simulink model "linearizzazione_feedback"  (R2022b)
settings: Solver=VariableStepAuto  StartTime=0.0  StopTime=30  FixedStep=0.01  RelTol=1e-3
settings Model: Creator=alexi  LastModifiedBy=alexi

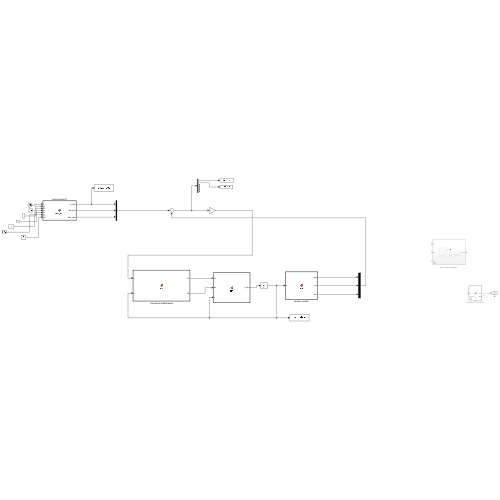
[thumbnail: Simulink's stored preview of the top-level diagram]
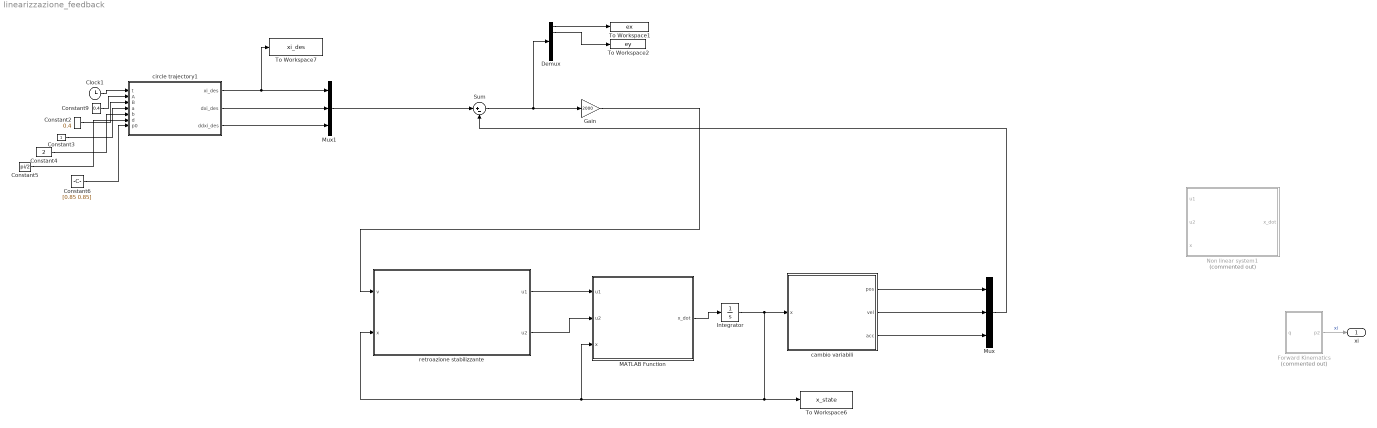
== system linearizzazione_feedback ==
  Clock1 : Clock
  Constant2 : Constant  Value=0.4
  Constant3 : Constant
  Constant4 : Constant  Value=2
  Constant5 : Constant  Value=pi/2
  Constant6 : Constant  Value=[0.85 0.85]
  Constant9 : Constant  Value=0.4
  Demux : Demux  Outputs=6
  Forward Kinematics : MATLAB Function  Commented=on  TreatAsAtomicUnit=on
  Gain : Gain  Gain=2000
  Integrator : Integrator  InitialCondition=[0.25 0.25 0 0 0.25 0.25]'
  MATLAB Function : MATLAB Function  TreatAsAtomicUnit=on
  Mux : Mux  Inputs=3
  Mux1 : Mux  Inputs=3
  Non linear system1 : Subsystem  Commented=on
  Sum : Sum  Inputs=|+-
  To Workspace1 : ToWorkspace  VariableName=ex  SaveFormat=Timeseries  SampleTime=-1
  To Workspace2 : ToWorkspace  VariableName=ey  SaveFormat=Timeseries  SampleTime=-1
  To Workspace6 : ToWorkspace  VariableName=x_state  SaveFormat=Timeseries  SampleTime=-1
  To Workspace7 : ToWorkspace  VariableName=xi_des  SaveFormat=Timeseries  SampleTime=-1
  cambio variabili : MATLAB Function  TreatAsAtomicUnit=on
  circle trajectory1 : MATLAB Function  TreatAsAtomicUnit=on
  retroazione stabilizzante : MATLAB Function  TreatAsAtomicUnit=on
  xi : Outport
  wires:
  Forward Kinematics/1(p2) -> xi/1  "xi"
  Constant4/1 -> circle trajectory1/5(b)
  Constant5/1 -> circle trajectory1/6(d)
  Constant2/1 -> circle trajectory1/3(B)
  Clock1/1 -> circle trajectory1/1(t)
  Constant6/1 -> circle trajectory1/7(p0)
  Constant3/1 -> circle trajectory1/4(a)
  Constant9/1 -> circle trajectory1/2(A)
  Integrator/1 -> MATLAB Function/3(x), retroazione stabilizzante/2(x), To Workspace6/1, cambio variabili/1(x)
  retroazione stabilizzante/1(u1) -> MATLAB Function/1(u1)
  retroazione stabilizzante/2(u2) -> MATLAB Function/2(u2)
  MATLAB Function/1(x_dot) -> Integrator/1
  cambio variabili/1(pos) -> Mux/1
  cambio variabili/2(vel) -> Mux/2
  cambio variabili/3(acc) -> Mux/3
  circle trajectory1/1(xi_des) -> To Workspace7/1, Mux1/1
  circle trajectory1/2(dxi_des) -> Mux1/2
  circle trajectory1/3(ddxi_des) -> Mux1/3
  Mux1/1 -> Sum/1
  Mux/1 -> Sum/2
  Sum/1 -> Demux/1, Gain/1
  Gain/1 -> retroazione stabilizzante/1(v)
  Demux/1 -> To Workspace1/1
  Demux/2 -> To Workspace2/1

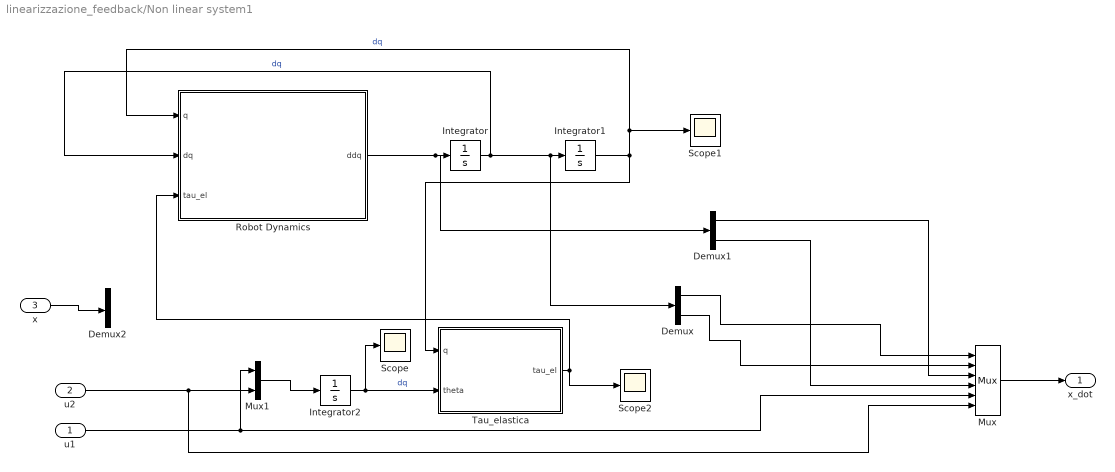
== system linearizzazione_feedback/Non linear system1 ==
  u1 : Inport
  u2 : Inport  Port=2
  x : Inport  Port=3
  Demux : Demux  Outputs=2
  Demux1 : Demux  Outputs=2
  Demux2 : Demux  Outputs=6
  Integrator : Integrator  InitialCondition=[0.25,0.25]'
  Integrator1 : Integrator  InitialCondition=[0.25,0.25]'
  Integrator2 : Integrator  InitialCondition=[0.25 0.25]'
  Mux : Mux  Inputs=6
  Mux1 : Mux  Inputs=2
  Robot Dynamics : MATLAB Function  TreatAsAtomicUnit=on
  Scope : Scope
  Scope1 : Scope
  Scope2 : Scope
  Tau_elastica : Subsystem
  x_dot : Outport
  wires:
  Integrator1/1 -> Tau_elastica/1(q), Scope1/1, Robot Dynamics/1(q)  "dq"
  Integrator/1 -> Robot Dynamics/2(dq), Demux/1, Integrator1/1  "dq"
  Tau_elastica/1(tau_el) -> Scope2/1, Robot Dynamics/3(tau_el)
  Robot Dynamics/1(ddq) -> Demux1/1, Integrator/1
  Demux/1 -> Mux/1
  Demux/2 -> Mux/2
  Demux1/1 -> Mux/3
  Demux1/2 -> Mux/4
  Integrator2/1 -> Scope/1, Tau_elastica/2(theta)  "dq"
  Mux/1 -> x_dot/1
  u1/1 -> Mux1/1, Mux/5
  u2/1 -> Mux1/2, Mux/6
  Mux1/1 -> Integrator2/1
  x/1 -> Demux2/1

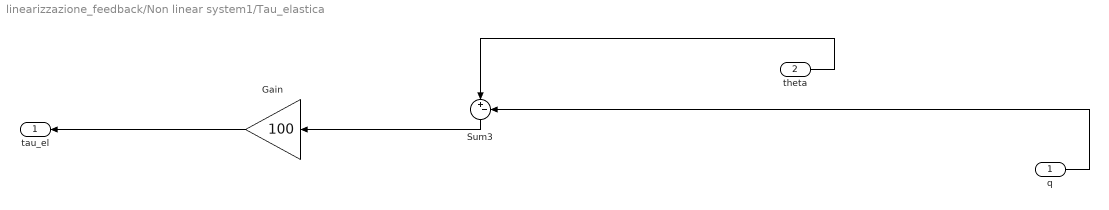
== system linearizzazione_feedback/Non linear system1/Tau_elastica ==
  q : Inport
  theta : Inport  Port=2
  Gain : Gain  Gain=100
  Sum3 : Sum  Inputs=|+-
  tau_el : Outport
  wires:
  Sum3/1 -> Gain/1
  q/1 -> Sum3/2
  Gain/1 -> tau_el/1
  theta/1 -> Sum3/1

== matlab function linearizzazione_feedback/cambio variabili ==
  data: x input; pos output; vel output; acc output
function [pos,vel,acc]= fcn(x)
a1 = 1;
a2 = 1;
k = 10;

q1 = x(1);
q2 = x(2);
dq1 = x(3);
dq2 = x(4);
theta1 = x(5);
theta2 = x(6);

q = [q1;q2];
dq = [dq1;dq2];
theta = [theta1;theta2];
B = RR_mass_matrix(q);
C = RR_coriolis_matrix(q,dq);
G = RR_gravity_vector(q);

% inversa_b = inv(B);
% B11G1 = inversa_b(1,1)*G(1);
% B12G2 = inversa_b(1,2)*G(2);
% B21G1 = inversa_b(2,1)*G(1);
% B22G2 = inversa_b(2,2)*G(2);
% 
% B11C11 = inversa_b(1,1)*C(1,1);
% B12C21 = inversa_b(1,2)*C(2,1);
% B11C12 = inversa_b(1,1)*C(1,2);
% B12C22 = inversa_b(1,2)*C(2,2);
%  
% B21C11 = inversa_b(2,1)*C(1,1);
% B22C21 = inversa_b(2,2)*C(2,1);
% B21C12 = inversa_b(2,1)*C(1,2);
% B22C22 = inversa_b(2,2)*C(2,2);
% 
% b1_1 = inversa_b(1,1);
% b1_2 = inversa_b(1,2);
% b2_1 = inversa_b(2,1);
% b2_2 = inversa_b(2,2);
% 
% c1_1 = C(1,1);
% c1_2 = C(1,2);
% c2_1 = C(2,1);
% c2_2 = C(2,2);
% 
% g1 = G(1);
% g2 = G(2);



% MG1 = MG(1);
% MG2 = MG(2);
% MC = inv(B)*C;
% MC1 = MC(1,1)+MC(1,2);
% MC2 = MC(2,1)+MC(2,2);
% inv = inv(B);
% B1 = inv(1,1) + inv(1,2);
% B2 = inv(2,1) + inv

z1 = a1*cos(q1)+a2*cos(q1+q2); %posizione in x
z2 = -sin(q1)*dq1 - sin(q1+q2)*(dq1+dq2); %derivata prima
%z3 = sin(q1 + q2)*(b1_1*g1 + b1_2*g2 + b2_1*g1 + b2_2*g2 + dq1*(b1_1*c1_1 + b1_2*c2_1) + dq2*(b1_1*c1_2 + b1_2*c2_2) + dq1*(b2_1*c1_1 + b2_2*c2_1) + dq2*(b2_1*c1_2 + b2_2*c2_2) + b1_1*k*(q1 - theta1) + b1_2*k*(q2 - theta2) + b2_1*k*(q1 - theta1) + b2_2*k*(q2 - theta2)) - cos(q1 + q2)*(dq1 + dq2)^2 + sin(q1)*(b1_1*g1 + b1_2*g2 + dq1*(b1_1*c1_1 + b1_2*c2_1) + dq2*(b1_1*c1_2 + b1_2*c2_2) + b1_1*k*(q1 - theta1) + b1_2*k*(q2 - theta2)) - cos(q1)*dq1^2;
z3 = sin(q1)*(dq1*((6*sin(q2)*dq2)/(9*cos(q2)^2 - 16) + (3*sin(q2)*dq1*(3*cos(q2) + 2))/(9*cos(q2)^2 - 16)) - (12*((2943*cos(q1))/200 + (981*cos(q1 + q2))/200))/(9*cos(q2)^2 - 16) - (12*k*(q1 - theta1))/(9*cos(q2)^2 - 16) + (2943*cos(q1 + q2)*(3*cos(q2) + 2))/(100*(9*cos(q2)^2 - 16)) + (6*k*(3*cos(q2) + 2)*(q2 - theta2))/(9*cos(q2)^2 - 16) + (6*sin(q2)*dq2*(dq1 + dq2))/(9*cos(q2)^2 - 16)) - cos(q1 + q2)*(dq1 + dq2)^2 - sin(q1 + q2)*((12*((2943*cos(q1))/200 + (981*cos(q1 + q2))/200))/(9*cos(q2)^2 - 16) - dq1*((6*sin(q2)*dq2)/(9*cos(q2)^2 - 16) + (3*sin(q2)*dq1*(3*cos(q2) + 2))/(9*cos(q2)^2 - 16)) + dq1*((3*sin(q2)*dq2*(3*cos(q2) + 2))/(9*cos(q2)^2 - 16) + (6*sin(q2)*dq1*(3*cos(q2) + 5))/(9*cos(q2)^2 - 16)) + (12*k*(q1 - theta1))/(9*cos(q2)^2 - 16) - (6*(3*cos(q2) + 2)*((2943*cos(q1))/200 + (981*cos(q1 + q2))/200))/(9*cos(q2)^2 - 16) - (2943*cos(q1 + q2)*(3*cos(q2) + 2))/(100*(9*cos(q2)^2 - 16)) + (2943*cos(q1 + q2)*(3*cos(q2) + 5))/(50*(9*cos(q2)^2 - 16)) - (6*k*(3*cos(q2) + 2)*(q1 - theta1))/(9*cos(q2)^2 - 16) - (6*k*(3*cos(q2) + 2)*(q2 - theta2))/(9*cos(q2)^2 - 16) + (12*k*(3*cos(q2) + 5)*(q2 - theta2))/(9*cos(q2)^2 - 16) - (6*sin(q2)*dq2*(dq1 + dq2))/(9*cos(q2)^2 - 16) + (3*sin(q2)*dq2*(3*cos(q2) + 2)*(dq1 + dq2))/(9*cos(q2)^2 - 16)) - cos(q1)*dq1^2;

z4 =  a1*sin(q1)+a2*sin(q1+q2); %posizione in y
z5 = cos(q1)*dq1 + cos(q1+q2)*(dq1+dq2);
%z6 = - cos(q1 + q2)*(b1_1*g1 + b1_2*g2 + b2_1*g1 + b2_2*g2 + dq1*(b1_1*c1_1 + b1_2*c2_1) + dq2*(b1_1*c1_2 + b1_2*c2_2) + dq1*(b2_1*c1_1 + b2_2*c2_1) + dq2*(b2_1*c1_2 + b2_2*c2_2) + b1_1*k*(q1 - theta1) + b1_2*k*(q2 - theta2) + b2_1*k*(q1 - theta1) + b2_2*k*(q2 - theta2)) - sin(q1 + q2)*(dq1 + dq2)^2 - cos(q1)*(b1_1*g1 + b1_2*g2 + dq1*(b1_1*c1_1 + b1_2*c2_1) + dq2*(b1_1*c1_2 + b1_2*c2_2) + b1_1*k*(q1 - theta1) + b1_2*k*(q2 - theta2)) - sin(q1)*dq1^2;
z6 = cos(q1 + q2)*((12*((2943*cos(q1))/200 + (981*cos(q1 + q2))/200))/(9*cos(q2)^2 - 16) - dq1*((6*sin(q2)*dq2)/(9*cos(q2)^2 - 16) + (3*sin(q2)*dq1*(3*cos(q2) + 2))/(9*cos(q2)^2 - 16)) + dq1*((3*sin(q2)*dq2*(3*cos(q2) + 2))/(9*cos(q2)^2 - 16) + (6*sin(q2)*dq1*(3*cos(q2) + 5))/(9*cos(q2)^2 - 16)) + (12*k*(q1 - theta1))/(9*cos(q2)^2 - 16) - (6*(3*cos(q2) + 2)*((2943*cos(q1))/200 + (981*cos(q1 + q2))/200))/(9*cos(q2)^2 - 16) - (2943*cos(q1 + q2)*(3*cos(q2) + 2))/(100*(9*cos(q2)^2 - 16)) + (2943*cos(q1 + q2)*(3*cos(q2) + 5))/(50*(9*cos(q2)^2 - 16)) - (6*k*(3*cos(q2) + 2)*(q1 - theta1))/(9*cos(q2)^2 - 16) - (6*k*(3*cos(q2) + 2)*(q2 - theta2))/(9*cos(q2)^2 - 16) + (12*k*(3*cos(q2) + 5)*(q2 - theta2))/(9*cos(q2)^2 - 16) - (6*sin(q2)*dq2*(dq1 + dq2))/(9*cos(q2)^2 - 16) + (3*sin(q2)*dq2*(3*cos(q2) + 2)*(dq1 + dq2))/(9*cos(q2)^2 - 16)) - cos(q1)*(dq1*((6*sin(q2)*dq2)/(9*cos(q2)^2 - 16) + (3*sin(q2)*dq1*(3*cos(q2) + 2))/(9*cos(q2)^2 - 16)) - (12*((2943*cos(q1))/200 + (981*cos(q1 + q2))/200))/(9*cos(q2)^2 - 16) - (12*k*(q1 - theta1))/(9*cos(q2)^2 - 16) + (2943*cos(q1 + q2)*(3*cos(q2) + 2))/(100*(9*cos(q2)^2 - 16)) + (6*k*(3*cos(q2) + 2)*(q2 - theta2))/(9*cos(q2)^2 - 16) + (6*sin(q2)*dq2*(dq1 + dq2))/(9*cos(q2)^2 - 16)) - sin(q1)*dq1^2 - sin(q1 + q2)*(dq1 + dq2)^2;
pos = [z1;z4];
vel = [z2;z5];
acc = [z3;z6];

== matlab function linearizzazione_feedback/retroazione stabilizzante ==
  data: v input; u1 output; x input; u2 output
function [u1,u2]= fcn(v,x)
k = 10;
q1 = x(1);
q2 = x(2);
dq1 = x(3);
dq2 = x(4);
theta1 = x(5);
theta2 = x(6);

q = [q1;q2];
dq = [dq1;dq2];
B = RR_mass_matrix(q);
C = RR_coriolis_matrix(q,dq);
G = RR_gravity_vector(q);

inversa_b = inv(B);
B11G1 = inversa_b(1,1)*G(1);
B12G2 = inversa_b(1,2)*G(2);
B21G1 = inversa_b(2,1)*G(1);
B22G2 = inversa_b(2,2)*G(2);

B11C11 = inversa_b(1,1)*C(1,1);
B12C21 = inversa_b(1,2)*C(2,1);
B11C12 = inversa_b(1,1)*C(1,2);
B12C22 = inversa_b(1,2)*C(2,2);
 
B21C11 = inversa_b(2,1)*C(1,1);
B22C21 = inversa_b(2,2)*C(2,1);
B21C12 = inversa_b(2,1)*C(1,2);
B22C22 = inversa_b(2,2)*C(2,2);

b1_1 = inversa_b(1,1);
b1_2 = inversa_b(1,2);
b2_1 = inversa_b(2,1);
b2_2 = inversa_b(2,2);

c1_1 = C(1,1);
c1_2 = C(1,2);
c2_1 = C(2,1);
c2_2 = C(2,2);

g1 = G(1);
g2 = G(2);

% x_dtheta1 = - sin(q1 + q2)*(b1_1*k + b2_1*k) - b1_1*k*sin(q1);
% x_dtheta2 = - sin(q1 + q2)*(b1_2*k + b2_2*k) - b1_2*k*sin(q1);
% y_dtheta1 = cos(q1 + q2)*(b1_1*k + b2_1*k) + b1_1*k*cos(q1);
% y_dtheta2 = cos(q1 + q2)*(b1_2*k + b2_2*k) + b1_2*k*cos(q1);

x_dtheta1 = sin(q1 + q2)*((12*k)/(9*cos(q2)^2 - 16) - (6*k*(3*cos(q2) + 2))/(9*cos(q2)^2 - 16)) + (12*k*sin(q1))/(9*cos(q2)^2 - 16);
x_dtheta2 = - sin(q1 + q2)*((6*k*(3*cos(q2) + 2))/(9*cos(q2)^2 - 16) - (12*k*(3*cos(q2) + 5))/(9*cos(q2)^2 - 16)) - (6*k*sin(q1)*(3*cos(q2) + 2))/(9*cos(q2)^2 - 16);
y_dtheta1 = - cos(q1 + q2)*((12*k)/(9*cos(q2)^2 - 16) - (6*k*(3*cos(q2) + 2))/(9*cos(q2)^2 - 16)) - (12*k*cos(q1))/(9*cos(q2)^2 - 16);
y_dtheta2 = cos(q1 + q2)*((6*k*(3*cos(q2) + 2))/(9*cos(q2)^2 - 16) - (12*k*(3*cos(q2) + 5))/(9*cos(q2)^2 - 16)) + (6*k*cos(q1)*(3*cos(q2) + 2))/(9*cos(q2)^2 - 16);

E = [x_dtheta1 x_dtheta2; y_dtheta1 y_dtheta2];
%f_x = sin(q1 + q2)*(dq1 + dq2)^3 - sin(q1)*((b1_1*c1_1 + b1_2*c2_1)*(b1_1*g1 + b1_2*g2 + dq1*(b1_1*c1_1 + b1_2*c2_1) + dq2*(b1_1*c1_2 + b1_2*c2_2) + b1_1*k*(q1 - theta1) + b1_2*k*(q2 - theta2)) + (b1_1*c1_2 + b1_2*c2_2)*(b2_1*g1 + b2_2*g2 + dq1*(b2_1*c1_1 + b2_2*c2_1) + dq2*(b2_1*c1_2 + b2_2*c2_2) + b2_1*k*(q1 - theta1) + b2_2*k*(q2 - theta2)) - b1_1*k*(dq1) - b1_2*k*(dq2)) - sin(q1 + q2)*((b1_1*c1_1 + b1_2*c2_1)*(b1_1*g1 + b1_2*g2 + dq1*(b1_1*c1_1 + b1_2*c2_1) + dq2*(b1_1*c1_2 + b1_2*c2_2) + b1_1*k*(q1 - theta1) + b1_2*k*(q2 - theta2)) + (b2_1*c1_1 + b2_2*c2_1)*(b1_1*g1 + b1_2*g2 + dq1*(b1_1*c1_1 + b1_2*c2_1) + dq2*(b1_1*c1_2 + b1_2*c2_2) + b1_1*k*(q1 - theta1) + b1_2*k*(q2 - theta2)) + (b1_1*c1_2 + b1_2*c2_2)*(b2_1*g1 + b2_2*g2 + dq1*(b2_1*c1_1 + b2_2*c2_1) + dq2*(b2_1*c1_2 + b2_2*c2_2) + b2_1*k*(q1 - theta1) + b2_2*k*(q2 - theta2)) + (b2_1*c1_2 + b2_2*c2_2)*(b2_1*g1 + b2_2*g2 + dq1*(b2_1*c1_1 + b2_2*c2_1) + dq2*(b2_1*c1_2 + b2_2*c2_2) + b2_1*k*(q1 - theta1) + b2_2*k*(q2 - theta2)) - b1_1*k*(dq1) - b1_2*k*(dq2) - b2_1*k*(dq1) - b2_2*k*(dq2)) + sin(q1)*dq1^3 + 3*cos(q1 + q2)*(dq1 + dq2)*(b1_1*g1 + b1_2*g2 + b2_1*g1 + b2_2*g2 + dq1*(b1_1*c1_1 + b1_2*c2_1) + dq2*(b1_1*c1_2 + b1_2*c2_2) + dq1*(b2_1*c1_1 + b2_2*c2_1) + dq2*(b2_1*c1_2 + b2_2*c2_2) + b1_1*k*(q1 - theta1) + b1_2*k*(q2 - theta2) + b2_1*k*(q1 - theta1) + b2_2*k*(q2 - theta2)) + 3*cos(q1)*dq1*(b1_1*g1 + b1_2*g2 + dq1*(b1_1*c1_1 + b1_2*c2_1) + dq2*(b1_1*c1_2 + b1_2*c2_2) + b1_1*k*(q1 - theta1) + b1_2*k*(q2 - theta2));
%f_y = cos(q1)*((b1_1*c1_1 + b1_2*c2_1)*(b1_1*g1 + b1_2*g2 + dq1*(b1_1*c1_1 + b1_2*c2_1) + dq2*(b1_1*c1_2 + b1_2*c2_2) + b1_1*k*(q1 - theta1) + b1_2*k*(q2 - theta2)) + (b1_1*c1_2 + b1_2*c2_2)*(b2_1*g1 + b2_2*g2 + dq1*(b2_1*c1_1 + b2_2*c2_1) + dq2*(b2_1*c1_2 + b2_2*c2_2) + b2_1*k*(q1 - theta1) + b2_2*k*(q2 - theta2)) - b1_1*k*(dq1) - b1_2*k*(dq2)) - cos(q1 + q2)*(dq1 + dq2)^3 + cos(q1 + q2)*((b1_1*c1_1 + b1_2*c2_1)*(b1_1*g1 + b1_2*g2 + dq1*(b1_1*c1_1 + b1_2*c2_1) + dq2*(b1_1*c1_2 + b1_2*c2_2) + b1_1*k*(q1 - theta1) + b1_2*k*(q2 - theta2)) + (b2_1*c1_1 + b2_2*c2_1)*(b1_1*g1 + b1_2*g2 + dq1*(b1_1*c1_1 + b1_2*c2_1) + dq2*(b1_1*c1_2 + b1_2*c2_2) + b1_1*k*(q1 - theta1) + b1_2*k*(q2 - theta2)) + (b1_1*c1_2 + b1_2*c2_2)*(b2_1*g1 + b2_2*g2 + dq1*(b2_1*c1_1 + b2_2*c2_1) + dq2*(b2_1*c1_2 + b2_2*c2_2) + b2_1*k*(q1 - theta1) + b2_2*k*(q2 - theta2)) + (b2_1*c1_2 + b2_2*c2_2)*(b2_1*g1 + b2_2*g2 + dq1*(b2_1*c1_1 + b2_2*c2_1) + dq2*(b2_1*c1_2 + b2_2*c2_2) + b2_1*k*(q1 - theta1) + b2_2*k*(q2 - theta2)) - b1_1*k*(dq1) - b1_2*k*(dq2) - b2_1*k*(dq1) - b2_2*k*(dq2)) - cos(q1)*dq1^3 + 3*sin(q1 + q2)*(dq1 + dq2)*(b1_1*g1 + b1_2*g2 + b2_1*g1 + b2_2*g2 + dq1*(b1_1*c1_1 + b1_2*c2_1) + dq2*(b1_1*c1_2 + b1_2*c2_2) + dq1*(b2_1*c1_1 + b2_2*c2_1) + dq2*(b2_1*c1_2 + b2_2*c2_2) + b1_1*k*(q1 - theta1) + b1_2*k*(q2 - theta2) + b2_1*k*(q1 - theta1) + b2_2*k*(q2 - theta2)) + 3*sin(q1)*dq1*(b1_1*g1 + b1_2*g2 + dq1*(b1_1*c1_1 + b1_2*c2_1) + dq2*(b1_1*c1_2 + b1_2*c2_2) + b1_1*k*(q1 - theta1) + b1_2*k*(q2 - theta2));
f_x = sin(q1 + q2)*(dq1 + dq2)^3 + sin(q1 + q2)*((12*((981*sin(q1 + q2)*(dq1 + dq2))/200 + (2943*sin(q1)*dq1)/200))/(9*cos(q2)^2 - 16) - ((6*sin(q2)*dq2)/(9*cos(q2)^2 - 16) + (3*sin(q2)*dq1*(3*cos(q2) + 2))/(9*cos(q2)^2 - 16))*(dq1*((6*sin(q2)*dq2)/(9*cos(q2)^2 - 16) + (3*sin(q2)*dq1*(3*cos(q2) + 2))/(9*cos(q2)^2 - 16)) - (12*((2943*cos(q1))/200 + (981*cos(q1 + q2))/200))/(9*cos(q2)^2 - 16) - (12*k*(q1 - theta1))/(9*cos(q2)^2 - 16) + (2943*cos(q1 + q2)*(3*cos(q2) + 2))/(100*(9*cos(q2)^2 - 16)) + (6*k*(3*cos(q2) + 2)*(q2 - theta2))/(9*cos(q2)^2 - 16) + (6*sin(q2)*dq2*(dq1 + dq2))/(9*cos(q2)^2 - 16)) + dq1*((6*cos(q2)*dq2^2)/(9*cos(q2)^2 - 16) + (6*sin(q2)*(dq1*((3*sin(q2)*dq2*(3*cos(q2) + 2))/(9*cos(q2)^2 - 16) + (6*sin(q2)*dq1*(3*cos(q2) + 5))/(9*cos(q2)^2 - 16)) - (6*(3*cos(q2) + 2)*((2943*cos(q1))/200 + (981*cos(q1 + q2))/200))/(9*cos(q2)^2 - 16) + (2943*cos(q1 + q2)*(3*cos(q2) + 5))/(50*(9*cos(q2)^2 - 16)) - (6*k*(3*cos(q2) + 2)*(q1 - theta1))/(9*cos(q2)^2 - 16) + (12*k*(3*cos(q2) + 5)*(q2 - theta2))/(9*cos(q2)^2 - 16) + (3*sin(q2)*dq2*(3*cos(q2) + 2)*(dq1 + dq2))/(9*cos(q2)^2 - 16)))/(9*cos(q2)^2 - 16) + (108*cos(q2)*sin(q2)^2*dq2^2)/(9*cos(q2)^2 - 16)^2 - (9*sin(q2)^2*dq1*dq2)/(9*cos(q2)^2 - 16) - (3*sin(q2)*(3*cos(q2) + 2)*(dq1*((6*sin(q2)*dq2)/(9*cos(q2)^2 - 16) + (3*sin(q2)*dq1*(3*cos(q2) + 2))/(9*cos(q2)^2 - 16)) - (12*((2943*cos(q1))/200 + (981*cos(q1 + q2))/200))/(9*cos(q2)^2 - 16) - (12*k*(q1 - theta1))/(9*cos(q2)^2 - 16) + (2943*cos(q1 + q2)*(3*cos(q2) + 2))/(100*(9*cos(q2)^2 - 16)) + (6*k*(3*cos(q2) + 2)*(q2 - theta2))/(9*cos(q2)^2 - 16) + (6*sin(q2)*dq2*(dq1 + dq2))/(9*cos(q2)^2 - 16)))/(9*cos(q2)^2 - 16) + (3*cos(q2)*dq1*dq2*(3*cos(q2) + 2))/(9*cos(q2)^2 - 16) + (54*cos(q2)*sin(q2)^2*dq1*dq2*(3*cos(q2) + 2))/(9*cos(q2)^2 - 16)^2) + ((3*sin(q2)*dq2*(3*cos(q2) + 2))/(9*cos(q2)^2 - 16) + (6*sin(q2)*dq1*(3*cos(q2) + 5))/(9*cos(q2)^2 - 16))*(dq1*((6*sin(q2)*dq2)/(9*cos(q2)^2 - 16) + (3*sin(q2)*dq1*(3*cos(q2) + 2))/(9*cos(q2)^2 - 16)) - (12*((2943*cos(q1))/200 + (981*cos(q1 + q2))/200))/(9*cos(q2)^2 - 16) - (12*k*(q1 - theta1))/(9*cos(q2)^2 - 16) + (2943*cos(q1 + q2)*(3*cos(q2) + 2))/(100*(9*cos(q2)^2 - 16)) + (6*k*(3*cos(q2) + 2)*(q2 - theta2))/(9*cos(q2)^2 - 16) + (6*sin(q2)*dq2*(dq1 + dq2))/(9*cos(q2)^2 - 16)) - dq1*((3*cos(q2)*dq2^2*(3*cos(q2) + 2))/(9*cos(q2)^2 - 16) - (18*sin(q2)^2*dq1*dq2)/(9*cos(q2)^2 - 16) - (6*sin(q2)*(3*cos(q2) + 5)*(dq1*((6*sin(q2)*dq2)/(9*cos(q2)^2 - 16) + (3*sin(q2)*dq1*(3*cos(q2) + 2))/(9*cos(q2)^2 - 16)) - (12*((2943*cos(q1))/200 + (981*cos(q1 + q2))/200))/(9*cos(q2)^2 - 16) - (12*k*(q1 - theta1))/(9*cos(q2)^2 - 16) + (2943*cos(q1 + q2)*(3*cos(q2) + 2))/(100*(9*cos(q2)^2 - 16)) + (6*k*(3*cos(q2) + 2)*(q2 - theta2))/(9*cos(q2)^2 - 16) + (6*sin(q2)*dq2*(dq1 + dq2))/(9*cos(q2)^2 - 16)))/(9*cos(q2)^2 - 16) - (9*sin(q2)^2*dq2^2)/(9*cos(q2)^2 - 16) + (3*sin(q2)*(3*cos(q2) + 2)*(dq1*((3*sin(q2)*dq2*(3*cos(q2) + 2))/(9*cos(q2)^2 - 16) + (6*sin(q2)*dq1*(3*cos(q2) + 5))/(9*cos(q2)^2 - 16)) - (6*(3*cos(q2) + 2)*((2943*cos(q1))/200 + (981*cos(q1 + q2))/200))/(9*cos(q2)^2 - 16) + (2943*cos(q1 + q2)*(3*cos(q2) + 5))/(50*(9*cos(q2)^2 - 16)) - (6*k*(3*cos(q2) + 2)*(q1 - theta1))/(9*cos(q2)^2 - 16) + (12*k*(3*cos(q2) + 5)*(q2 - theta2))/(9*cos(q2)^2 - 16) + (3*sin(q2)*dq2*(3*cos(q2) + 2)*(dq1 + dq2))/(9*cos(q2)^2 - 16)))/(9*cos(q2)^2 - 16) + (6*cos(q2)*dq1*dq2*(3*cos(q2) + 5))/(9*cos(q2)^2 - 16) + (54*cos(q2)*sin(q2)^2*dq2^2*(3*cos(q2) + 2))/(9*cos(q2)^2 - 16)^2 + (108*cos(q2)*sin(q2)^2*dq1*dq2*(3*cos(q2) + 5))/(9*cos(q2)^2 - 16)^2) - (12*k*(dq1))/(9*cos(q2)^2 - 16) - (6*(3*cos(q2) + 2)*((981*sin(q1 + q2)*(dq1 + dq2))/200 + (2943*sin(q1)*dq1)/200))/(9*cos(q2)^2 - 16) + (6*k*(3*cos(q2) + 2)*(dq1))/(9*cos(q2)^2 - 16) + (6*k*(3*cos(q2) + 2)*(dq2))/(9*cos(q2)^2 - 16) - (12*k*(3*cos(q2) + 5)*(dq2))/(9*cos(q2)^2 - 16) + (9*sin(q2)^2*dq2^2*(dq1 + dq2))/(9*cos(q2)^2 - 16) - (18*sin(q2)*dq2*((2943*cos(q1))/200 + (981*cos(q1 + q2))/200))/(9*cos(q2)^2 - 16) + (6*sin(q2)*dq2*((12*((2943*cos(q1))/200 + (981*cos(q1 + q2))/200))/(9*cos(q2)^2 - 16) - dq1*((6*sin(q2)*dq2)/(9*cos(q2)^2 - 16) + (3*sin(q2)*dq1*(3*cos(q2) + 2))/(9*cos(q2)^2 - 16)) + dq1*((3*sin(q2)*dq2*(3*cos(q2) + 2))/(9*cos(q2)^2 - 16) + (6*sin(q2)*dq1*(3*cos(q2) + 5))/(9*cos(q2)^2 - 16)) + (12*k*(q1 - theta1))/(9*cos(q2)^2 - 16) - (6*(3*cos(q2) + 2)*((2943*cos(q1))/200 + (981*cos(q1 + q2))/200))/(9*cos(q2)^2 - 16) - (2943*cos(q1 + q2)*(3*cos(q2) + 2))/(100*(9*cos(q2)^2 - 16)) + (2943*cos(q1 + q2)*(3*cos(q2) + 5))/(50*(9*cos(q2)^2 - 16)) - (6*k*(3*cos(q2) + 2)*(q1 - theta1))/(9*cos(q2)^2 - 16) - (6*k*(3*cos(q2) + 2)*(q2 - theta2))/(9*cos(q2)^2 - 16) + (12*k*(3*cos(q2) + 5)*(q2 - theta2))/(9*cos(q2)^2 - 16) - (6*sin(q2)*dq2*(dq1 + dq2))/(9*cos(q2)^2 - 16) + (3*sin(q2)*dq2*(3*cos(q2) + 2)*(dq1 + dq2))/(9*cos(q2)^2 - 16)))/(9*cos(q2)^2 - 16) + (6*cos(q2)*dq2^2*(dq1 + dq2))/(9*cos(q2)^2 - 16) + (6*sin(q2)*(dq1 + dq2)*(dq1*((3*sin(q2)*dq2*(3*cos(q2) + 2))/(9*cos(q2)^2 - 16) + (6*sin(q2)*dq1*(3*cos(q2) + 5))/(9*cos(q2)^2 - 16)) - (6*(3*cos(q2) + 2)*((2943*cos(q1))/200 + (981*cos(q1 + q2))/200))/(9*cos(q2)^2 - 16) + (2943*cos(q1 + q2)*(3*cos(q2) + 5))/(50*(9*cos(q2)^2 - 16)) - (6*k*(3*cos(q2) + 2)*(q1 - theta1))/(9*cos(q2)^2 - 16) + (12*k*(3*cos(q2) + 5)*(q2 - theta2))/(9*cos(q2)^2 - 16) + (3*sin(q2)*dq2*(3*cos(q2) + 2)*(dq1 + dq2))/(9*cos(q2)^2 - 16)))/(9*cos(q2)^2 - 16) - (2943*sin(q1 + q2)*(3*cos(q2) + 2)*(dq1 + dq2))/(100*(9*cos(q2)^2 - 16)) + (2943*sin(q1 + q2)*(3*cos(q2) + 5)*(dq1 + dq2))/(50*(9*cos(q2)^2 - 16)) + (8829*sin(q2)*cos(q1 + q2)*dq2)/(100*(9*cos(q2)^2 - 16)) - (18*k*sin(q2)*dq2*(q1 - theta1))/(9*cos(q2)^2 - 16) + (18*k*sin(q2)*dq2*(q2 - theta2))/(9*cos(q2)^2 - 16) - (3*sin(q2)*dq2*(3*cos(q2) + 2)*((12*((2943*cos(q1))/200 + (981*cos(q1 + q2))/200))/(9*cos(q2)^2 - 16) - dq1*((6*sin(q2)*dq2)/(9*cos(q2)^2 - 16) + (3*sin(q2)*dq1*(3*cos(q2) + 2))/(9*cos(q2)^2 - 16)) + dq1*((3*sin(q2)*dq2*(3*cos(q2) + 2))/(9*cos(q2)^2 - 16) + (6*sin(q2)*dq1*(3*cos(q2) + 5))/(9*cos(q2)^2 - 16)) + (12*k*(q1 - theta1))/(9*cos(q2)^2 - 16) - (6*(3*cos(q2) + 2)*((2943*cos(q1))/200 + (981*cos(q1 + q2))/200))/(9*cos(q2)^2 - 16) - (2943*cos(q1 + q2)*(3*cos(q2) + 2))/(100*(9*cos(q2)^2 - 16)) + (2943*cos(q1 + q2)*(3*cos(q2) + 5))/(50*(9*cos(q2)^2 - 16)) - (6*k*(3*cos(q2) + 2)*(q1 - theta1))/(9*cos(q2)^2 - 16) - (6*k*(3*cos(q2) + 2)*(q2 - theta2))/(9*cos(q2)^2 - 16) + (12*k*(3*cos(q2) + 5)*(q2 - theta2))/(9*cos(q2)^2 - 16) - (6*sin(q2)*dq2*(dq1 + dq2))/(9*cos(q2)^2 - 16) + (3*sin(q2)*dq2*(3*cos(q2) + 2)*(dq1 + dq2))/(9*cos(q2)^2 - 16)))/(9*cos(q2)^2 - 16) + (108*cos(q2)*sin(q2)^2*dq2^2*(dq1 + dq2))/(9*cos(q2)^2 - 16)^2 - (216*cos(q2)*sin(q2)*dq2*((2943*cos(q1))/200 + (981*cos(q1 + q2))/200))/(9*cos(q2)^2 - 16)^2 - (3*cos(q2)*dq2^2*(3*cos(q2) + 2)*(dq1 + dq2))/(9*cos(q2)^2 - 16) - (3*sin(q2)*(3*cos(q2) + 2)*(dq1 + dq2)*(dq1*((3*sin(q2)*dq2*(3*cos(q2) + 2))/(9*cos(q2)^2 - 16) + (6*sin(q2)*dq1*(3*cos(q2) + 5))/(9*cos(q2)^2 - 16)) - (6*(3*cos(q2) + 2)*((2943*cos(q1))/200 + (981*cos(q1 + q2))/200))/(9*cos(q2)^2 - 16) + (2943*cos(q1 + q2)*(3*cos(q2) + 5))/(50*(9*cos(q2)^2 - 16)) - (6*k*(3*cos(q2) + 2)*(q1 - theta1))/(9*cos(q2)^2 - 16) + (12*k*(3*cos(q2) + 5)*(q2 - theta2))/(9*cos(q2)^2 - 16) + (3*sin(q2)*dq2*(3*cos(q2) + 2)*(dq1 + dq2))/(9*cos(q2)^2 - 16)))/(9*cos(q2)^2 - 16) + (26487*cos(q2)*sin(q2)*cos(q1 + q2)*dq2*(3*cos(q2) + 2))/(50*(9*cos(q2)^2 - 16)^2) - (26487*cos(q2)*sin(q2)*cos(q1 + q2)*dq2*(3*cos(q2) + 5))/(25*(9*cos(q2)^2 - 16)^2) - (54*cos(q2)*sin(q2)^2*dq2^2*(3*cos(q2) + 2)*(dq1 + dq2))/(9*cos(q2)^2 - 16)^2 - (216*k*cos(q2)*sin(q2)*dq2*(q1 - theta1))/(9*cos(q2)^2 - 16)^2 + (108*cos(q2)*sin(q2)*dq2*(3*cos(q2) + 2)*((2943*cos(q1))/200 + (981*cos(q1 + q2))/200))/(9*cos(q2)^2 - 16)^2 + (108*k*cos(q2)*sin(q2)*dq2*(3*cos(q2) + 2)*(q1 - theta1))/(9*cos(q2)^2 - 16)^2 + (108*k*cos(q2)*sin(q2)*dq2*(3*cos(q2) + 2)*(q2 - theta2))/(9*cos(q2)^2 - 16)^2 - (216*k*cos(q2)*sin(q2)*dq2*(3*cos(q2) + 5)*(q2 - theta2))/(9*cos(q2)^2 - 16)^2) + sin(q1)*((12*((981*sin(q1 + q2)*(dq1 + dq2))/200 + (2943*sin(q1)*dq1)/200))/(9*cos(q2)^2 - 16) - ((6*sin(q2)*dq2)/(9*cos(q2)^2 - 16) + (3*sin(q2)*dq1*(3*cos(q2) + 2))/(9*cos(q2)^2 - 16))*(dq1*((6*sin(q2)*dq2)/(9*cos(q2)^2 - 16) + (3*sin(q2)*dq1*(3*cos(q2) + 2))/(9*cos(q2)^2 - 16)) - (12*((2943*cos(q1))/200 + (981*cos(q1 + q2))/200))/(9*cos(q2)^2 - 16) - (12*k*(q1 - theta1))/(9*cos(q2)^2 - 16) + (2943*cos(q1 + q2)*(3*cos(q2) + 2))/(100*(9*cos(q2)^2 - 16)) + (6*k*(3*cos(q2) + 2)*(q2 - theta2))/(9*cos(q2)^2 - 16) + (6*sin(q2)*dq2*(dq1 + dq2))/(9*cos(q2)^2 - 16)) + dq1*((6*cos(q2)*dq2^2)/(9*cos(q2)^2 - 16) + (6*sin(q2)*(dq1*((3*sin(q2)*dq2*(3*cos(q2) + 2))/(9*cos(q2)^2 - 16) + (6*sin(q2)*dq1*(3*cos(q2) + 5))/(9*cos(q2)^2 - 16)) - (6*(3*cos(q2) + 2)*((2943*cos(q1))/200 + (981*cos(q1 + q2))/200))/(9*cos(q2)^2 - 16) + (2943*cos(q1 + q2)*(3*cos(q2) + 5))/(50*(9*cos(q2)^2 - 16)) - (6*k*(3*cos(q2) + 2)*(q1 - theta1))/(9*cos(q2)^2 - 16) + (12*k*(3*cos(q2) + 5)*(q2 - theta2))/(9*cos(q2)^2 - 16) + (3*sin(q2)*dq2*(3*cos(q2) + 2)*(dq1 + dq2))/(9*cos(q2)^2 - 16)))/(9*cos(q2)^2 - 16) + (108*cos(q2)*sin(q2)^2*dq2^2)/(9*cos(q2)^2 - 16)^2 - (9*sin(q2)^2*dq1*dq2)/(9*cos(q2)^2 - 16) - (3*sin(q2)*(3*cos(q2) + 2)*(dq1*((6*sin(q2)*dq2)/(9*cos(q2)^2 - 16) + (3*sin(q2)*dq1*(3*cos(q2) + 2))/(9*cos(q2)^2 - 16)) - (12*((2943*cos(q1))/200 + (981*cos(q1 + q2))/200))/(9*cos(q2)^2 - 16) - (12*k*(q1 - theta1))/(9*cos(q2)^2 - 16) + (2943*cos(q1 + q2)*(3*cos(q2) + 2))/(100*(9*cos(q2)^2 - 16)) + (6*k*(3*cos(q2) + 2)*(q2 - theta2))/(9*cos(q2)^2 - 16) + (6*sin(q2)*dq2*(dq1 + dq2))/(9*cos(q2)^2 - 16)))/(9*cos(q2)^2 - 16) + (3*cos(q2)*dq1*dq2*(3*cos(q2) + 2))/(9*cos(q2)^2 - 16) + (54*cos(q2)*sin(q2)^2*dq1*dq2*(3*cos(q2) + 2))/(9*cos(q2)^2 - 16)^2) - (12*k*(dq1))/(9*cos(q2)^2 - 16) + (6*k*(3*cos(q2) + 2)*(dq2))/(9*cos(q2)^2 - 16) + (6*sin(q2)*dq2*((12*((2943*cos(q1))/200 + (981*cos(q1 + q2))/200))/(9*cos(q2)^2 - 16) - dq1*((6*sin(q2)*dq2)/(9*cos(q2)^2 - 16) + (3*sin(q2)*dq1*(3*cos(q2) + 2))/(9*cos(q2)^2 - 16)) + dq1*((3*sin(q2)*dq2*(3*cos(q2) + 2))/(9*cos(q2)^2 - 16) + (6*sin(q2)*dq1*(3*cos(q2) + 5))/(9*cos(q2)^2 - 16)) + (12*k*(q1 - theta1))/(9*cos(q2)^2 - 16) - (6*(3*cos(q2) + 2)*((2943*cos(q1))/200 + (981*cos(q1 + q2))/200))/(9*cos(q2)^2 - 16) - (2943*cos(q1 + q2)*(3*cos(q2) + 2))/(100*(9*cos(q2)^2 - 16)) + (2943*cos(q1 + q2)*(3*cos(q2) + 5))/(50*(9*cos(q2)^2 - 16)) - (6*k*(3*cos(q2) + 2)*(q1 - theta1))/(9*cos(q2)^2 - 16) - (6*k*(3*cos(q2) + 2)*(q2 - theta2))/(9*cos(q2)^2 - 16) + (12*k*(3*cos(q2) + 5)*(q2 - theta2))/(9*cos(q2)^2 - 16) - (6*sin(q2)*dq2*(dq1 + dq2))/(9*cos(q2)^2 - 16) + (3*sin(q2)*dq2*(3*cos(q2) + 2)*(dq1 + dq2))/(9*cos(q2)^2 - 16)))/(9*cos(q2)^2 - 16) + (6*cos(q2)*dq2^2*(dq1 + dq2))/(9*cos(q2)^2 - 16) + (6*sin(q2)*(dq1 + dq2)*(dq1*((3*sin(q2)*dq2*(3*cos(q2) + 2))/(9*cos(q2)^2 - 16) + (6*sin(q2)*dq1*(3*cos(q2) + 5))/(9*cos(q2)^2 - 16)) - (6*(3*cos(q2) + 2)*((2943*cos(q1))/200 + (981*cos(q1 + q2))/200))/(9*cos(q2)^2 - 16) + (2943*cos(q1 + q2)*(3*cos(q2) + 5))/(50*(9*cos(q2)^2 - 16)) - (6*k*(3*cos(q2) + 2)*(q1 - theta1))/(9*cos(q2)^2 - 16) + (12*k*(3*cos(q2) + 5)*(q2 - theta2))/(9*cos(q2)^2 - 16) + (3*sin(q2)*dq2*(3*cos(q2) + 2)*(dq1 + dq2))/(9*cos(q2)^2 - 16)))/(9*cos(q2)^2 - 16) - (2943*sin(q1 + q2)*(3*cos(q2) + 2)*(dq1 + dq2))/(100*(9*cos(q2)^2 - 16)) - (8829*sin(q2)*cos(q1 + q2)*dq2)/(100*(9*cos(q2)^2 - 16)) - (18*k*sin(q2)*dq2*(q2 - theta2))/(9*cos(q2)^2 - 16) + (108*cos(q2)*sin(q2)^2*dq2^2*(dq1 + dq2))/(9*cos(q2)^2 - 16)^2 - (216*cos(q2)*sin(q2)*dq2*((2943*cos(q1))/200 + (981*cos(q1 + q2))/200))/(9*cos(q2)^2 - 16)^2 + (26487*cos(q2)*sin(q2)*cos(q1 + q2)*dq2*(3*cos(q2) + 2))/(50*(9*cos(q2)^2 - 16)^2) - (216*k*cos(q2)*sin(q2)*dq2*(q1 - theta1))/(9*cos(q2)^2 - 16)^2 + (108*k*cos(q2)*sin(q2)*dq2*(3*cos(q2) + 2)*(q2 - theta2))/(9*cos(q2)^2 - 16)^2) + sin(q1)*dq1^3 - 3*cos(q1 + q2)*(dq1 + dq2)*((12*((2943*cos(q1))/200 + (981*cos(q1 + q2))/200))/(9*cos(q2)^2 - 16) - dq1*((6*sin(q2)*dq2)/(9*cos(q2)^2 - 16) + (3*sin(q2)*dq1*(3*cos(q2) + 2))/(9*cos(q2)^2 - 16)) + dq1*((3*sin(q2)*dq2*(3*cos(q2) + 2))/(9*cos(q2)^2 - 16) + (6*sin(q2)*dq1*(3*cos(q2) + 5))/(9*cos(q2)^2 - 16)) + (12*k*(q1 - theta1))/(9*cos(q2)^2 - 16) - (6*(3*cos(q2) + 2)*((2943*cos(q1))/200 + (981*cos(q1 + q2))/200))/(9*cos(q2)^2 - 16) - (2943*cos(q1 + q2)*(3*cos(q2) + 2))/(100*(9*cos(q2)^2 - 16)) + (2943*cos(q1 + q2)*(3*cos(q2) + 5))/(50*(9*cos(q2)^2 - 16)) - (6*k*(3*cos(q2) + 2)*(q1 - theta1))/(9*cos(q2)^2 - 16) - (6*k*(3*cos(q2) + 2)*(q2 - theta2))/(9*cos(q2)^2 - 16) + (12*k*(3*cos(q2) + 5)*(q2 - theta2))/(9*cos(q2)^2 - 16) - (6*sin(q2)*dq2*(dq1 + dq2))/(9*cos(q2)^2 - 16) + (3*sin(q2)*dq2*(3*cos(q2) + 2)*(dq1 + dq2))/(9*cos(q2)^2 - 16)) + 3*cos(q1)*dq1*(dq1*((6*sin(q2)*dq2)/(9*cos(q2)^2 - 16) + (3*sin(q2)*dq1*(3*cos(q2) + 2))/(9*cos(q2)^2 - 16)) - (12*((2943*cos(q1))/200 + (981*cos(q1 + q2))/200))/(9*cos(q2)^2 - 16) - (12*k*(q1 - theta1))/(9*cos(q2)^2 - 16) + (2943*cos(q1 + q2)*(3*cos(q2) + 2))/(100*(9*cos(q2)^2 - 16)) + (6*k*(3*cos(q2) + 2)*(q2 - theta2))/(9*cos(q2)^2 - 16) + (6*sin(q2)*dq2*(dq1 + dq2))/(9*cos(q2)^2 - 16));
f_y = 3*sin(q1)*dq1*(dq1*((6*sin(q2)*dq2)/(9*cos(q2)^2 - 16) + (3*sin(q2)*dq1*(3*cos(q2) + 2))/(9*cos(q2)^2 - 16)) - (12*((2943*cos(q1))/200 + (981*cos(q1 + q2))/200))/(9*cos(q2)^2 - 16) - (12*k*(q1 - theta1))/(9*cos(q2)^2 - 16) + (2943*cos(q1 + q2)*(3*cos(q2) + 2))/(100*(9*cos(q2)^2 - 16)) + (6*k*(3*cos(q2) + 2)*(q2 - theta2))/(9*cos(q2)^2 - 16) + (6*sin(q2)*dq2*(dq1 + dq2))/(9*cos(q2)^2 - 16)) - cos(q1 + q2)*((12*((981*sin(q1 + q2)*(dq1 + dq2))/200 + (2943*sin(q1)*dq1)/200))/(9*cos(q2)^2 - 16) - ((6*sin(q2)*dq2)/(9*cos(q2)^2 - 16) + (3*sin(q2)*dq1*(3*cos(q2) + 2))/(9*cos(q2)^2 - 16))*(dq1*((6*sin(q2)*dq2)/(9*cos(q2)^2 - 16) + (3*sin(q2)*dq1*(3*cos(q2) + 2))/(9*cos(q2)^2 - 16)) - (12*((2943*cos(q1))/200 + (981*cos(q1 + q2))/200))/(9*cos(q2)^2 - 16) - (12*k*(q1 - theta1))/(9*cos(q2)^2 - 16) + (2943*cos(q1 + q2)*(3*cos(q2) + 2))/(100*(9*cos(q2)^2 - 16)) + (6*k*(3*cos(q2) + 2)*(q2 - theta2))/(9*cos(q2)^2 - 16) + (6*sin(q2)*dq2*(dq1 + dq2))/(9*cos(q2)^2 - 16)) + dq1*((6*cos(q2)*dq2^2)/(9*cos(q2)^2 - 16) + (6*sin(q2)*(dq1*((3*sin(q2)*dq2*(3*cos(q2) + 2))/(9*cos(q2)^2 - 16) + (6*sin(q2)*dq1*(3*cos(q2) + 5))/(9*cos(q2)^2 - 16)) - (6*(3*cos(q2) + 2)*((2943*cos(q1))/200 + (981*cos(q1 + q2))/200))/(9*cos(q2)^2 - 16) + (2943*cos(q1 + q2)*(3*cos(q2) + 5))/(50*(9*cos(q2)^2 - 16)) - (6*k*(3*cos(q2) + 2)*(q1 - theta1))/(9*cos(q2)^2 - 16) + (12*k*(3*cos(q2) + 5)*(q2 - theta2))/(9*cos(q2)^2 - 16) + (3*sin(q2)*dq2*(3*cos(q2) + 2)*(dq1 + dq2))/(9*cos(q2)^2 - 16)))/(9*cos(q2)^2 - 16) + (108*cos(q2)*sin(q2)^2*dq2^2)/(9*cos(q2)^2 - 16)^2 - (9*sin(q2)^2*dq1*dq2)/(9*cos(q2)^2 - 16) - (3*sin(q2)*(3*cos(q2) + 2)*(dq1*((6*sin(q2)*dq2)/(9*cos(q2)^2 - 16) + (3*sin(q2)*dq1*(3*cos(q2) + 2))/(9*cos(q2)^2 - 16)) - (12*((2943*cos(q1))/200 + (981*cos(q1 + q2))/200))/(9*cos(q2)^2 - 16) - (12*k*(q1 - theta1))/(9*cos(q2)^2 - 16) + (2943*cos(q1 + q2)*(3*cos(q2) + 2))/(100*(9*cos(q2)^2 - 16)) + (6*k*(3*cos(q2) + 2)*(q2 - theta2))/(9*cos(q2)^2 - 16) + (6*sin(q2)*dq2*(dq1 + dq2))/(9*cos(q2)^2 - 16)))/(9*cos(q2)^2 - 16) + (3*cos(q2)*dq1*dq2*(3*cos(q2) + 2))/(9*cos(q2)^2 - 16) + (54*cos(q2)*sin(q2)^2*dq1*dq2*(3*cos(q2) + 2))/(9*cos(q2)^2 - 16)^2) + ((3*sin(q2)*dq2*(3*cos(q2) + 2))/(9*cos(q2)^2 - 16) + (6*sin(q2)*dq1*(3*cos(q2) + 5))/(9*cos(q2)^2 - 16))*(dq1*((6*sin(q2)*dq2)/(9*cos(q2)^2 - 16) + (3*sin(q2)*dq1*(3*cos(q2) + 2))/(9*cos(q2)^2 - 16)) - (12*((2943*cos(q1))/200 + (981*cos(q1 + q2))/200))/(9*cos(q2)^2 - 16) - (12*k*(q1 - theta1))/(9*cos(q2)^2 - 16) + (2943*cos(q1 + q2)*(3*cos(q2) + 2))/(100*(9*cos(q2)^2 - 16)) + (6*k*(3*cos(q2) + 2)*(q2 - theta2))/(9*cos(q2)^2 - 16) + (6*sin(q2)*dq2*(dq1 + dq2))/(9*cos(q2)^2 - 16)) - dq1*((3*cos(q2)*dq2^2*(3*cos(q2) + 2))/(9*cos(q2)^2 - 16) - (18*sin(q2)^2*dq1*dq2)/(9*cos(q2)^2 - 16) - (6*sin(q2)*(3*cos(q2) + 5)*(dq1*((6*sin(q2)*dq2)/(9*cos(q2)^2 - 16) + (3*sin(q2)*dq1*(3*cos(q2) + 2))/(9*cos(q2)^2 - 16)) - (12*((2943*cos(q1))/200 + (981*cos(q1 + q2))/200))/(9*cos(q2)^2 - 16) - (12*k*(q1 - theta1))/(9*cos(q2)^2 - 16) + (2943*cos(q1 + q2)*(3*cos(q2) + 2))/(100*(9*cos(q2)^2 - 16)) + (6*k*(3*cos(q2) + 2)*(q2 - theta2))/(9*cos(q2)^2 - 16) + (6*sin(q2)*dq2*(dq1 + dq2))/(9*cos(q2)^2 - 16)))/(9*cos(q2)^2 - 16) - (9*sin(q2)^2*dq2^2)/(9*cos(q2)^2 - 16) + (3*sin(q2)*(3*cos(q2) + 2)*(dq1*((3*sin(q2)*dq2*(3*cos(q2) + 2))/(9*cos(q2)^2 - 16) + (6*sin(q2)*dq1*(3*cos(q2) + 5))/(9*cos(q2)^2 - 16)) - (6*(3*cos(q2) + 2)*((2943*cos(q1))/200 + (981*cos(q1 + q2))/200))/(9*cos(q2)^2 - 16) + (2943*cos(q1 + q2)*(3*cos(q2) + 5))/(50*(9*cos(q2)^2 - 16)) - (6*k*(3*cos(q2) + 2)*(q1 - theta1))/(9*cos(q2)^2 - 16) + (12*k*(3*cos(q2) + 5)*(q2 - theta2))/(9*cos(q2)^2 - 16) + (3*sin(q2)*dq2*(3*cos(q2) + 2)*(dq1 + dq2))/(9*cos(q2)^2 - 16)))/(9*cos(q2)^2 - 16) + (6*cos(q2)*dq1*dq2*(3*cos(q2) + 5))/(9*cos(q2)^2 - 16) + (54*cos(q2)*sin(q2)^2*dq2^2*(3*cos(q2) + 2))/(9*cos(q2)^2 - 16)^2 + (108*cos(q2)*sin(q2)^2*dq1*dq2*(3*cos(q2) + 5))/(9*cos(q2)^2 - 16)^2) - (12*k*(dq1))/(9*cos(q2)^2 - 16) - (6*(3*cos(q2) + 2)*((981*sin(q1 + q2)*(dq1 + dq2))/200 + (2943*sin(q1)*dq1)/200))/(9*cos(q2)^2 - 16) + (6*k*(3*cos(q2) + 2)*(dq1))/(9*cos(q2)^2 - 16) + (6*k*(3*cos(q2) + 2)*(dq2))/(9*cos(q2)^2 - 16) - (12*k*(3*cos(q2) + 5)*(dq2))/(9*cos(q2)^2 - 16) + (9*sin(q2)^2*dq2^2*(dq1 + dq2))/(9*cos(q2)^2 - 16) - (18*sin(q2)*dq2*((2943*cos(q1))/200 + (981*cos(q1 + q2))/200))/(9*cos(q2)^2 - 16) + (6*sin(q2)*dq2*((12*((2943*cos(q1))/200 + (981*cos(q1 + q2))/200))/(9*cos(q2)^2 - 16) - dq1*((6*sin(q2)*dq2)/(9*cos(q2)^2 - 16) + (3*sin(q2)*dq1*(3*cos(q2) + 2))/(9*cos(q2)^2 - 16)) + dq1*((3*sin(q2)*dq2*(3*cos(q2) + 2))/(9*cos(q2)^2 - 16) + (6*sin(q2)*dq1*(3*cos(q2) + 5))/(9*cos(q2)^2 - 16)) + (12*k*(q1 - theta1))/(9*cos(q2)^2 - 16) - (6*(3*cos(q2) + 2)*((2943*cos(q1))/200 + (981*cos(q1 + q2))/200))/(9*cos(q2)^2 - 16) - (2943*cos(q1 + q2)*(3*cos(q2) + 2))/(100*(9*cos(q2)^2 - 16)) + (2943*cos(q1 + q2)*(3*cos(q2) + 5))/(50*(9*cos(q2)^2 - 16)) - (6*k*(3*cos(q2) + 2)*(q1 - theta1))/(9*cos(q2)^2 - 16) - (6*k*(3*cos(q2) + 2)*(q2 - theta2))/(9*cos(q2)^2 - 16) + (12*k*(3*cos(q2) + 5)*(q2 - theta2))/(9*cos(q2)^2 - 16) - (6*sin(q2)*dq2*(dq1 + dq2))/(9*cos(q2)^2 - 16) + (3*sin(q2)*dq2*(3*cos(q2) + 2)*(dq1 + dq2))/(9*cos(q2)^2 - 16)))/(9*cos(q2)^2 - 16) + (6*cos(q2)*dq2^2*(dq1 + dq2))/(9*cos(q2)^2 - 16) + (6*sin(q2)*(dq1 + dq2)*(dq1*((3*sin(q2)*dq2*(3*cos(q2) + 2))/(9*cos(q2)^2 - 16) + (6*sin(q2)*dq1*(3*cos(q2) + 5))/(9*cos(q2)^2 - 16)) - (6*(3*cos(q2) + 2)*((2943*cos(q1))/200 + (981*cos(q1 + q2))/200))/(9*cos(q2)^2 - 16) + (2943*cos(q1 + q2)*(3*cos(q2) + 5))/(50*(9*cos(q2)^2 - 16)) - (6*k*(3*cos(q2) + 2)*(q1 - theta1))/(9*cos(q2)^2 - 16) + (12*k*(3*cos(q2) + 5)*(q2 - theta2))/(9*cos(q2)^2 - 16) + (3*sin(q2)*dq2*(3*cos(q2) + 2)*(dq1 + dq2))/(9*cos(q2)^2 - 16)))/(9*cos(q2)^2 - 16) - (2943*sin(q1 + q2)*(3*cos(q2) + 2)*(dq1 + dq2))/(100*(9*cos(q2)^2 - 16)) + (2943*sin(q1 + q2)*(3*cos(q2) + 5)*(dq1 + dq2))/(50*(9*cos(q2)^2 - 16)) + (8829*sin(q2)*cos(q1 + q2)*dq2)/(100*(9*cos(q2)^2 - 16)) - (18*k*sin(q2)*dq2*(q1 - theta1))/(9*cos(q2)^2 - 16) + (18*k*sin(q2)*dq2*(q2 - theta2))/(9*cos(q2)^2 - 16) - (3*sin(q2)*dq2*(3*cos(q2) + 2)*((12*((2943*cos(q1))/200 + (981*cos(q1 + q2))/200))/(9*cos(q2)^2 - 16) - dq1*((6*sin(q2)*dq2)/(9*cos(q2)^2 - 16) + (3*sin(q2)*dq1*(3*cos(q2) + 2))/(9*cos(q2)^2 - 16)) + dq1*((3*sin(q2)*dq2*(3*cos(q2) + 2))/(9*cos(q2)^2 - 16) + (6*sin(q2)*dq1*(3*cos(q2) + 5))/(9*cos(q2)^2 - 16)) + (12*k*(q1 - theta1))/(9*cos(q2)^2 - 16) - (6*(3*cos(q2) + 2)*((2943*cos(q1))/200 + (981*cos(q1 + q2))/200))/(9*cos(q2)^2 - 16) - (2943*cos(q1 + q2)*(3*cos(q2) + 2))/(100*(9*cos(q2)^2 - 16)) + (2943*cos(q1 + q2)*(3*cos(q2) + 5))/(50*(9*cos(q2)^2 - 16)) - (6*k*(3*cos(q2) + 2)*(q1 - theta1))/(9*cos(q2)^2 - 16) - (6*k*(3*cos(q2) + 2)*(q2 - theta2))/(9*cos(q2)^2 - 16) + (12*k*(3*cos(q2) + 5)*(q2 - theta2))/(9*cos(q2)^2 - 16) - (6*sin(q2)*dq2*(dq1 + dq2))/(9*cos(q2)^2 - 16) + (3*sin(q2)*dq2*(3*cos(q2) + 2)*(dq1 + dq2))/(9*cos(q2)^2 - 16)))/(9*cos(q2)^2 - 16) + (108*cos(q2)*sin(q2)^2*dq2^2*(dq1 + dq2))/(9*cos(q2)^2 - 16)^2 - (216*cos(q2)*sin(q2)*dq2*((2943*cos(q1))/200 + (981*cos(q1 + q2))/200))/(9*cos(q2)^2 - 16)^2 - (3*cos(q2)*dq2^2*(3*cos(q2) + 2)*(dq1 + dq2))/(9*cos(q2)^2 - 16) - (3*sin(q2)*(3*cos(q2) + 2)*(dq1 + dq2)*(dq1*((3*sin(q2)*dq2*(3*cos(q2) + 2))/(9*cos(q2)^2 - 16) + (6*sin(q2)*dq1*(3*cos(q2) + 5))/(9*cos(q2)^2 - 16)) - (6*(3*cos(q2) + 2)*((2943*cos(q1))/200 + (981*cos(q1 + q2))/200))/(9*cos(q2)^2 - 16) + (2943*cos(q1 + q2)*(3*cos(q2) + 5))/(50*(9*cos(q2)^2 - 16)) - (6*k*(3*cos(q2) + 2)*(q1 - theta1))/(9*cos(q2)^2 - 16) + (12*k*(3*cos(q2) + 5)*(q2 - theta2))/(9*cos(q2)^2 - 16) + (3*sin(q2)*dq2*(3*cos(q2) + 2)*(dq1 + dq2))/(9*cos(q2)^2 - 16)))/(9*cos(q2)^2 - 16) + (26487*cos(q2)*sin(q2)*cos(q1 + q2)*dq2*(3*cos(q2) + 2))/(50*(9*cos(q2)^2 - 16)^2) - (26487*cos(q2)*sin(q2)*cos(q1 + q2)*dq2*(3*cos(q2) + 5))/(25*(9*cos(q2)^2 - 16)^2) - (54*cos(q2)*sin(q2)^2*dq2^2*(3*cos(q2) + 2)*(dq1 + dq2))/(9*cos(q2)^2 - 16)^2 - (216*k*cos(q2)*sin(q2)*dq2*(q1 - theta1))/(9*cos(q2)^2 - 16)^2 + (108*cos(q2)*sin(q2)*dq2*(3*cos(q2) + 2)*((2943*cos(q1))/200 + (981*cos(q1 + q2))/200))/(9*cos(q2)^2 - 16)^2 + (108*k*cos(q2)*sin(q2)*dq2*(3*cos(q2) + 2)*(q1 - theta1))/(9*cos(q2)^2 - 16)^2 + (108*k*cos(q2)*sin(q2)*dq2*(3*cos(q2) + 2)*(q2 - theta2))/(9*cos(q2)^2 - 16)^2 - (216*k*cos(q2)*sin(q2)*dq2*(3*cos(q2) + 5)*(q2 - theta2))/(9*cos(q2)^2 - 16)^2) - cos(q1)*((12*((981*sin(q1 + q2)*(dq1 + dq2))/200 + (2943*sin(q1)*dq1)/200))/(9*cos(q2)^2 - 16) - ((6*sin(q2)*dq2)/(9*cos(q2)^2 - 16) + (3*sin(q2)*dq1*(3*cos(q2) + 2))/(9*cos(q2)^2 - 16))*(dq1*((6*sin(q2)*dq2)/(9*cos(q2)^2 - 16) + (3*sin(q2)*dq1*(3*cos(q2) + 2))/(9*cos(q2)^2 - 16)) - (12*((2943*cos(q1))/200 + (981*cos(q1 + q2))/200))/(9*cos(q2)^2 - 16) - (12*k*(q1 - theta1))/(9*cos(q2)^2 - 16) + (2943*cos(q1 + q2)*(3*cos(q2) + 2))/(100*(9*cos(q2)^2 - 16)) + (6*k*(3*cos(q2) + 2)*(q2 - theta2))/(9*cos(q2)^2 - 16) + (6*sin(q2)*dq2*(dq1 + dq2))/(9*cos(q2)^2 - 16)) + dq1*((6*cos(q2)*dq2^2)/(9*cos(q2)^2 - 16) + (6*sin(q2)*(dq1*((3*sin(q2)*dq2*(3*cos(q2) + 2))/(9*cos(q2)^2 - 16) + (6*sin(q2)*dq1*(3*cos(q2) + 5))/(9*cos(q2)^2 - 16)) - (6*(3*cos(q2) + 2)*((2943*cos(q1))/200 + (981*cos(q1 + q2))/200))/(9*cos(q2)^2 - 16) + (2943*cos(q1 + q2)*(3*cos(q2) + 5))/(50*(9*cos(q2)^2 - 16)) - (6*k*(3*cos(q2) + 2)*(q1 - theta1))/(9*cos(q2)^2 - 16) + (12*k*(3*cos(q2) + 5)*(q2 - theta2))/(9*cos(q2)^2 - 16) + (3*sin(q2)*dq2*(3*cos(q2) + 2)*(dq1 + dq2))/(9*cos(q2)^2 - 16)))/(9*cos(q2)^2 - 16) + (108*cos(q2)*sin(q2)^2*dq2^2)/(9*cos(q2)^2 - 16)^2 - (9*sin(q2)^2*dq1*dq2)/(9*cos(q2)^2 - 16) - (3*sin(q2)*(3*cos(q2) + 2)*(dq1*((6*sin(q2)*dq2)/(9*cos(q2)^2 - 16) + (3*sin(q2)*dq1*(3*cos(q2) + 2))/(9*cos(q2)^2 - 16)) - (12*((2943*cos(q1))/200 + (981*cos(q1 + q2))/200))/(9*cos(q2)^2 - 16) - (12*k*(q1 - theta1))/(9*cos(q2)^2 - 16) + (2943*cos(q1 + q2)*(3*cos(q2) + 2))/(100*(9*cos(q2)^2 - 16)) + (6*k*(3*cos(q2) + 2)*(q2 - theta2))/(9*cos(q2)^2 - 16) + (6*sin(q2)*dq2*(dq1 + dq2))/(9*cos(q2)^2 - 16)))/(9*cos(q2)^2 - 16) + (3*cos(q2)*dq1*dq2*(3*cos(q2) + 2))/(9*cos(q2)^2 - 16) + (54*cos(q2)*sin(q2)^2*dq1*dq2*(3*cos(q2) + 2))/(9*cos(q2)^2 - 16)^2) - (12*k*(dq1))/(9*cos(q2)^2 - 16) + (6*k*(3*cos(q2) + 2)*(dq2))/(9*cos(q2)^2 - 16) + (6*sin(q2)*dq2*((12*((2943*cos(q1))/200 + (981*cos(q1 + q2))/200))/(9*cos(q2)^2 - 16) - dq1*((6*sin(q2)*dq2)/(9*cos(q2)^2 - 16) + (3*sin(q2)*dq1*(3*cos(q2) + 2))/(9*cos(q2)^2 - 16)) + dq1*((3*sin(q2)*dq2*(3*cos(q2) + 2))/(9*cos(q2)^2 - 16) + (6*sin(q2)*dq1*(3*cos(q2) + 5))/(9*cos(q2)^2 - 16)) + (12*k*(q1 - theta1))/(9*cos(q2)^2 - 16) - (6*(3*cos(q2) + 2)*((2943*cos(q1))/200 + (981*cos(q1 + q2))/200))/(9*cos(q2)^2 - 16) - (2943*cos(q1 + q2)*(3*cos(q2) + 2))/(100*(9*cos(q2)^2 - 16)) + (2943*cos(q1 + q2)*(3*cos(q2) + 5))/(50*(9*cos(q2)^2 - 16)) - (6*k*(3*cos(q2) + 2)*(q1 - theta1))/(9*cos(q2)^2 - 16) - (6*k*(3*cos(q2) + 2)*(q2 - theta2))/(9*cos(q2)^2 - 16) + (12*k*(3*cos(q2) + 5)*(q2 - theta2))/(9*cos(q2)^2 - 16) - (6*sin(q2)*dq2*(dq1 + dq2))/(9*cos(q2)^2 - 16) + (3*sin(q2)*dq2*(3*cos(q2) + 2)*(dq1 + dq2))/(9*cos(q2)^2 - 16)))/(9*cos(q2)^2 - 16) + (6*cos(q2)*dq2^2*(dq1 + dq2))/(9*cos(q2)^2 - 16) + (6*sin(q2)*(dq1 + dq2)*(dq1*((3*sin(q2)*dq2*(3*cos(q2) + 2))/(9*cos(q2)^2 - 16) + (6*sin(q2)*dq1*(3*cos(q2) + 5))/(9*cos(q2)^2 - 16)) - (6*(3*cos(q2) + 2)*((2943*cos(q1))/200 + (981*cos(q1 + q2))/200))/(9*cos(q2)^2 - 16) + (2943*cos(q1 + q2)*(3*cos(q2) + 5))/(50*(9*cos(q2)^2 - 16)) - (6*k*(3*cos(q2) + 2)*(q1 - theta1))/(9*cos(q2)^2 - 16) + (12*k*(3*cos(q2) + 5)*(q2 - theta2))/(9*cos(q2)^2 - 16) + (3*sin(q2)*dq2*(3*cos(q2) + 2)*(dq1 + dq2))/(9*cos(q2)^2 - 16)))/(9*cos(q2)^2 - 16) - (2943*sin(q1 + q2)*(3*cos(q2) + 2)*(dq1 + dq2))/(100*(9*cos(q2)^2 - 16)) - (8829*sin(q2)*cos(q1 + q2)*dq2)/(100*(9*cos(q2)^2 - 16)) - (18*k*sin(q2)*dq2*(q2 - theta2))/(9*cos(q2)^2 - 16) + (108*cos(q2)*sin(q2)^2*dq2^2*(dq1 + dq2))/(9*cos(q2)^2 - 16)^2 - (216*cos(q2)*sin(q2)*dq2*((2943*cos(q1))/200 + (981*cos(q1 + q2))/200))/(9*cos(q2)^2 - 16)^2 + (26487*cos(q2)*sin(q2)*cos(q1 + q2)*dq2*(3*cos(q2) + 2))/(50*(9*cos(q2)^2 - 16)^2) - (216*k*cos(q2)*sin(q2)*dq2*(q1 - theta1))/(9*cos(q2)^2 - 16)^2 + (108*k*cos(q2)*sin(q2)*dq2*(3*cos(q2) + 2)*(q2 - theta2))/(9*cos(q2)^2 - 16)^2) - cos(q1)*dq1^3 - 3*sin(q1 + q2)*(dq1 + dq2)*((12*((2943*cos(q1))/200 + (981*cos(q1 + q2))/200))/(9*cos(q2)^2 - 16) - dq1*((6*sin(q2)*dq2)/(9*cos(q2)^2 - 16) + (3*sin(q2)*dq1*(3*cos(q2) + 2))/(9*cos(q2)^2 - 16)) + dq1*((3*sin(q2)*dq2*(3*cos(q2) + 2))/(9*cos(q2)^2 - 16) + (6*sin(q2)*dq1*(3*cos(q2) + 5))/(9*cos(q2)^2 - 16)) + (12*k*(q1 - theta1))/(9*cos(q2)^2 - 16) - (6*(3*cos(q2) + 2)*((2943*cos(q1))/200 + (981*cos(q1 + q2))/200))/(9*cos(q2)^2 - 16) - (2943*cos(q1 + q2)*(3*cos(q2) + 2))/(100*(9*cos(q2)^2 - 16)) + (2943*cos(q1 + q2)*(3*cos(q2) + 5))/(50*(9*cos(q2)^2 - 16)) - (6*k*(3*cos(q2) + 2)*(q1 - theta1))/(9*cos(q2)^2 - 16) - (6*k*(3*cos(q2) + 2)*(q2 - theta2))/(9*cos(q2)^2 - 16) + (12*k*(3*cos(q2) + 5)*(q2 - theta2))/(9*cos(q2)^2 - 16) - (6*sin(q2)*dq2*(dq1 + dq2))/(9*cos(q2)^2 - 16) + (3*sin(q2)*dq2*(3*cos(q2) + 2)*(dq1 + dq2))/(9*cos(q2)^2 - 16)) - cos(q1 + q2)*(dq1 + dq2)^3;
F = [f_x;f_y];

vx = v(1) + v(3) + v(5);
vy = v(2) + v(4) + v(6);
o = [vx;vy];
%v = -dddp+o;
u = -inv(E)*F + inv(E)*o;
u1 = u(1);
u2 = u(2);
oppo = -pinv(E)*F;

== matlab function linearizzazione_feedback/circle trajectory1 ==
  data: t input; xi_des output; dxi_des output; A input; B input; a input; b input; d input; p0 input; ddxi_des output
function [xi_des, dxi_des, ddxi_des] = lissajous(t,A,B,a,b,d,p0)

xi_des = [A*sin(a*t+d); B*sin(b*t)] + p0;
dxi_des = [A*a*cos(a*t+d); B*b*cos(b*t)];
ddxi_des = [-A*a^2*sin(a*t+d); -B*b^2*sin(b*t)];

== matlab function linearizzazione_feedback/MATLAB Function ==
  data: u1 input; x_dot output; u2 input; x input
function x_dot  = fcn(u1,u2,x)
x1 = x(1);
x2 = x(2);
x3 = x(3);
x4 = x(4);
x5 = x(5);
x6 = x(6);
k = 10;

q = [x1;x2];
dq = [x3;x4];
B = RR_mass_matrix(q);
C = RR_coriolis_matrix(q,dq);
G = RR_gravity_vector(q);

theta = [x5;x6];
q = [x1;x2];
dq = [x3;x4];
q_ddot = inv(B)*k*(theta - q)- inv(B)*C*dq - inv(B)*G;

x1_dot = x3;
x2_dot = x4;
x3_dot = q_ddot(1);
x4_dot = q_ddot(2);
x5_dot = u1;
x6_dot = u2;
x_dot = [x1_dot;x2_dot;x3_dot;x4_dot;x5_dot;x6_dot];

== matlab function linearizzazione_feedback/Forward Kinematics ==
  data: q input; p2 output
function p2  = RR_forward_kinematics(q)

    q1 = q(1);
    q2 = q(2);

    a1 = 1;
    a2 = 1;

    p0 = [0;0];
    p1 = [a1*cos(q1); a1*sin(q1)];
    p2 = p1+[a2*cos(q1+q2);a2*sin(a1+q2)];
end

== matlab function linearizzazione_feedback/Non linear system1/Robot Dynamics ==
  data: q input; dq input; tau_el input; ddq output
function ddq = inverse_dynamics(q,dq, tau_el)

% Get dynamic matrices
B = RR_mass_matrix(q);
C = RR_coriolis_matrix(q,dq);
G = RR_gravity_vector(q);
ddq = pinv(B)*(tau_el - C*dq - G);
